simulink model "test"  (R2022a)
settings: Solver=VariableStepAuto  StartTime=0.0  StopTime=10.0  RelTol=1e-3
settings Model: Creator=radek  LastModifiedBy=radek

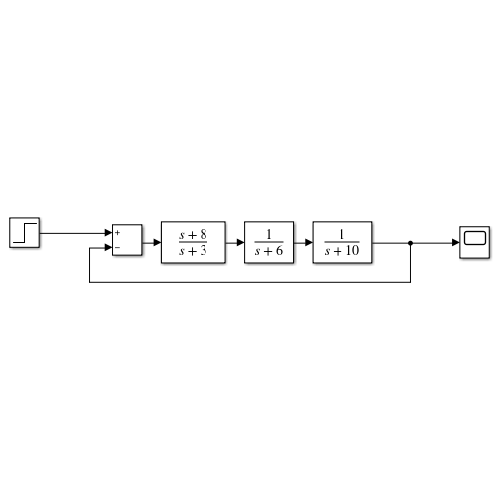
[thumbnail: Simulink's stored preview of the top-level diagram]
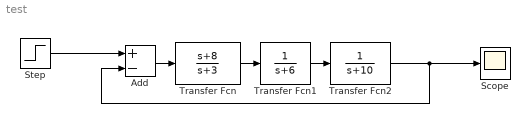
== system test ==
  Add : Sum  Inputs=+-
  Scope : Scope
  Step : Step  Time=0  SampleTime=0
  Transfer Fcn : TransferFcn  Numerator=[1 8]  Denominator=[1 3]
  Transfer Fcn1 : TransferFcn  Denominator=[1 6]
  Transfer Fcn2 : TransferFcn  Denominator=[1 10]
  wires:
  Step/1 -> Add/1
  Add/1 -> Transfer Fcn/1
  Transfer Fcn/1 -> Transfer Fcn1/1
  Transfer Fcn1/1 -> Transfer Fcn2/1
  Transfer Fcn2/1 -> Scope/1, Add/2
